simulink model "BAI1"  (Simulink 9.0)
settings: Solver=FixedStepAuto  StartTime=0.0  StopTime=20  FixedStep=0.01  RelTol=1e-3
undefined symbols (not defined in the file): A, B, C, L
libraries: simulink x2
settings Model: Creator=DELL  LastModifiedBy=DELL
settings DataIOCC: SaveFormat=Dataset
settings OptimizationCC: LifeSpan=auto
settings DebuggingCC: UnderspecifiedInitializationDetection=Simplified  MergeDetectMultiDrivingBlocksExec=error  SFUnexpectedBacktrackingDiag=error  SFNoUnconditionalDefaultTransitionDiag=error  SFExecutionAtInitializationDiag=warning
settings HardwareCC: ProdBitPerPointer=64  ProdBitPerSizeT=64  ProdBitPerPtrDiffT=64  ProdLargestAtomicFloat=Float  ProdIntDivRoundTo=Zero  ProdEndianess=LittleEndian  ProdWordSize=64  ProdHWDeviceType=Intel->x86-64 (Windows64)
settings ModelReferenceCC: PropagateSignalLabelsOutOfModel=on
settings CodeAppCC: StateflowObjectComments=off
settings GRTTargetCC: TargetLangStandard=C99 (ISO)
settings ConfigComp: CovMetricSettings=dwe  CovHtmlReporting=off  CovSaveCumulativeToWorkspaceVar=off  CovSaveSingleToWorkspaceVar=off  CovExternalEMLEnable=on

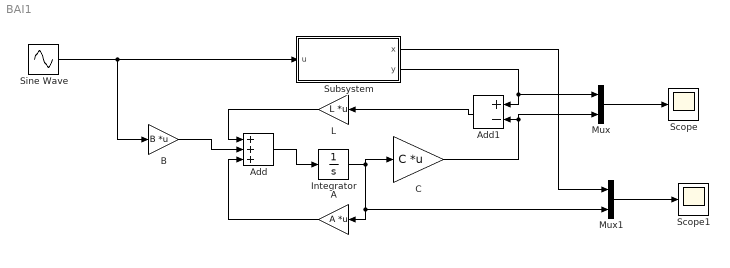
== system BAI1 ==
  A : Gain  Gain=A  Multiplication=Matrix(K*u) (u vector)
  Add : Sum  Inputs=+++
  Add1 : Sum  Inputs=+-
  B : Gain  Gain=B  Multiplication=Matrix(K*u) (u vector)
  C : Gain  Gain=C  Multiplication=Matrix(K*u) (u vector)
  Integrator : Integrator  InitialCondition=[0;0]
  "L " : Gain  Gain=L  Multiplication=Matrix(K*u) (u vector)
  Mux : Mux  Inputs=2
  Mux1 : Mux  Inputs=2
  Scope : Scope
  Scope1 : Scope
  Sine Wave : Sin  Frequency=2*pi*0.1  SampleTime=0
  Subsystem : Subsystem
  wires:
  Sine Wave/1 -> B/1, Subsystem/1(u)
  B/1 -> Add/2
  "L "/1 -> Add/1
  A/1 -> Add/3
  Add/1 -> Integrator/1
  Integrator/1 -> C/1, Mux1/2, A/1
  Add1/1 -> "L "/1
  Subsystem/2(y) -> Add1/1, Mux/1
  C/1 -> Mux/2, Add1/2
  Mux/1 -> Scope/1
  Mux1/1 -> Scope1/1
  Subsystem/1(x) -> Mux1/1

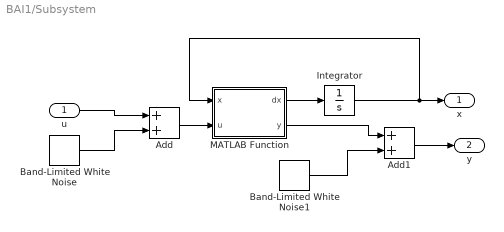
== system BAI1/Subsystem ==
  u : Inport
  Add : Sum
  Add1 : Sum
  Band-Limited White Noise : simulink/Sources/Band-Limited White Noise  Cov=[0.0001]  Ts=0.01  seed=[23341]
  Band-Limited White Noise1 : simulink/Sources/Band-Limited White Noise  Cov=[0.001]  Ts=0.01  seed=[23341]
  Integrator : Integrator  InitialCondition=[0.2;0.3]
  MATLAB Function : MATLAB Function  TreatAsAtomicUnit=on
  x : Outport
  y : Outport  Port=2
  wires:
  MATLAB Function/1(dx) -> Integrator/1
  Integrator/1 -> MATLAB Function/1(x), x/1
  u/1 -> Add/1
  Band-Limited White Noise/1 -> Add/2
  Add/1 -> MATLAB Function/2(u)
  Band-Limited White Noise1/1 -> Add1/2
  MATLAB Function/2(y) -> Add1/1
  Add1/1 -> y/1

== matlab function Subsystem/MATLAB Function ==
  data: x input double; dx output double; u input double; y output double
function [dx,y] = System1(x,u)
A=[0 1;-1 -2];
B=[0;1];
C=[1 0];
dx=A*x+B*u;
y = C*x;
